simulink model "Modelo_Red_Mitigación_final"  (R2019b)
settings: Solver=VariableStepAuto  StartTime=0.0  StopTime=2.5  RelTol=1e-3
InitFcn:
  | Ts=20e-6;
undefined symbols (not defined in the file): D1, Delta, Ion, Lithium
libraries: powerlib x371, powerlib_meascontrol x286, simulink x50, simulink_extras x20, electricdrivelib x16
(part 1 of 11)
settings Model: Creator=ASUS  LastModifiedBy=mance
settings SolverCC: AlgebraicLoopSolver=LineSearch

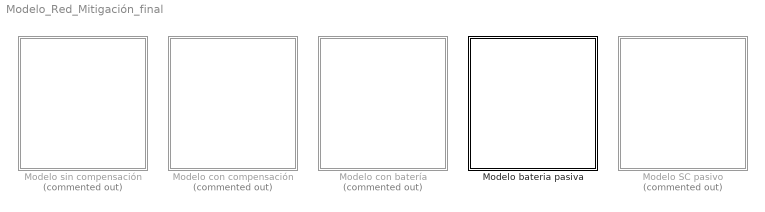
== system Modelo_Red_Mitigación_final ==
  Modelo SC pasivo : Subsystem  Commented=on
  Modelo bateria pasiva : Subsystem
  "Modelo con batería " : Subsystem  Commented=on
  Modelo con compensación : Subsystem  Commented=on
  Modelo sin compensación : Subsystem  Commented=on

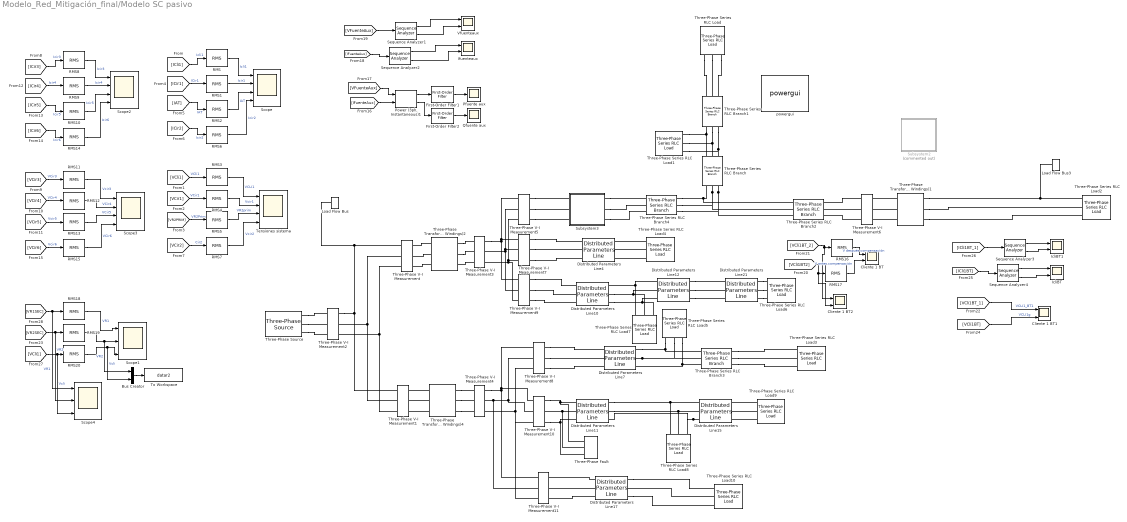
== system Modelo_Red_Mitigación_final/Modelo SC pasivo ==
  Bus Creator : BusCreator  Inputs=2
  Cliente 1 BT : Scope  NumInputPorts=2
  Cliente 1 BT1 : Scope  NumInputPorts=3
  Cliente 1 BT2 : Scope  NumInputPorts=2
  Distributed Parameters Line10 : powerlib/Elements/Distributed Parameters Line  Phases=3  Frequency=60  Resistance=[0.213 0.639]  Inductance=[0.78e-3 2.35e-3]  Capacitance=[15e-9 15e-9]  Length=3  x1=[-2e-05 2.82954479507891e-09 32197.4628123599 -19329.1003175042;-1e-05 2.80813823558566e-09 32270.1028326165 -19207.5816752081]  x2=[-2e-05 2.77830767246127e-09 31710.0647284196 -19350.9504482248;-1e-05 2.75705345961333e-09 31782.7905850361 -19231.2690937948]  x3=[-2e-05 -1.24111133051853e-11 -137.606557855475 265.255923665155;-1e-05 -1.24858274424735e-11 -138.605568913231 264.73527545555]  x4=[-2e-05 2.72589848097641e-11 416.943661034301 -435.06441838885;-1e-05 2.72249332713776e-11 418.580848519875 -433.489489926912]  x5=1.78115131305569e-05  V1=ones(3,3)  V2=ones(3,3)  I1=ones(3,3)  I2=ones(3,3)  nHarmo=1  Measurements=None
      settings: SourceProductName=Simscape Electrical
  Distributed Parameters Line11 : powerlib/Elements/Distributed Parameters Line  Phases=3  Frequency=60  Resistance=[0.269 0.807]  Inductance=[0.85e-3 2.56e-3]  Capacitance=[15e-9 15e-9]  Length=18  x1=[-0.00012 9.28558517205125e-09 31499.5304856781 -20459.5850295864;-0.00011 9.33622831118938e-09 31576.4372823811 -20340.6894905972;-0.0001 9.38673876185742e-09 31652.8953080157 -20221.5048653861;-9e-05 9.43711580619005e-09 31728.9034759441 -20102.0328478305;-8e-05 9.48735872821797e-09 31804.460705922 -19982.2751358921;-7e-05 9.53746681387805e-09 31879.565924114 -19862.2334315932;-6e-05 9.58743935102346e-09 31954.2180631086 -19741.9094409921;-5e-05 9.63727562943386e-09 32028.4160619336 -19621.304874159;-4e-05 9.68697494082539e-09 32102.1588660714 -19500.4214451518;-3e-05 9.73653657886085e-09 32175.4454274734 -19379.2608719915;-2e-05 9.78595983915965e-09 32248.2747045753 -19257.8248766382;-1e-05 9.83524401930785e-09 32320.645662312 -19136.1151849661]  x2=[-0.00012 7.5254042731239e-09 29691.2836160491 -20133.8764409861;-0.00011 7.57085579555663e-09 29766.9753728049 -20021.8001304674;-0.0001 7.61619971937037e-09 29842.2440749513 -19909.4392658505;-9e-05 7.6614354001276e-09 29917.0886527534 -19796.795444032;-8e-05 7.70656219492916e-09 29991.5080425041 -19683.87026593;-7e-05 7.75157946242343e-09 30065.5011865392 -19570.6653364611;-6e-05 7.79648656281536e-09 30139.0670332523 -19457.182264518;-5e-05 7.84128285787568e-09 30212.2045371099 -19343.4226629463;-4e-05 7.88596771094986e-09 30284.9126586661 -19229.3881485218;-3e-05 7.93054048696724e-09 30357.1903645776 -19115.0803419274;-2e-05 7.97500055245001e-09 30429.0366276182 -19000.50086773;-1e-05 8.01934727552222e-09 30500.4504266936 -18885.6513543576]  x3=[-0.00012 1.82517240735292e-11 9.27297529817065 123.366608204449;-0.00011 1.80056496454053e-11 8.80782934901758 123.400689758644;-0.0001 1.77593193171444e-11 8.34255822111328 123.43301751589;-9e-05 1.75127365896455e-11 7.87716852699037 123.463591016737;-8e-05 1.72659049673952e-11 7.41166688086653 123.492409826668;-7e-05 1.70188279584172e-11 6.94605989855056 123.519473536105;-6e-05 1.67715090742226e-11 6.48035419734828 123.544781760411;-5e-05 1.65239518297602e-11 6.01455639596856 123.568334139902;-4e-05 1.62761597433665e-11 5.5486731144292 123.590130339845;-3e-05 1.60281363367154e-11 5.08271097396287 123.610170050469;-2e-05 1.57798851347687e-11 4.616676596923 123.628452986965;-1e-05 1.55314096657253e-11 4.15057660668964 123.644978889491]  x4=[-0.00012 1.97670884628206e-11 241.846087556996 -294.396448705046;-0.00011 2.02416146680514e-11 242.954214808572 -293.482620581729;-0.0001 2.07158531951328e-11 244.058889142975 -292.564621420748;-9e-05 2.11897973040857e-11 245.160094860337 -291.642464268904;-8e-05 2.16634402591152e-11 246.257816310088 -290.71616223209;-7e-05 2.21367753287064e-11 247.352037891177 -289.78572847511;-6e-05 2.26097957857204e-11 248.442744052292 -288.851176221485;-5e-05 2.30824949074893e-11 249.529919292085 -287.912518753273;-4e-05 2.35548659759124e-11 250.613548159388 -286.969769410873;-3e-05 2.40269022775511e-11 251.693615253439 -286.022941592841;-2e-05 2.44985971037248e-11 252.770105224091 -285.072048755695;-1e-05 2.49699437506059e-11 253.84300277204 -284.117104413728]  x5=0.000111541920370774  V1=ones(3,3)  V2=ones(3,3)  I1=ones(3,3)  I2=ones(3,3)  nHarmo=1  Measurements=None
      settings: SourceProductName=Simscape Electrical
  Distributed Parameters Line12 : powerlib/Elements/Distributed Parameters Line  Phases=3  Frequency=60  Resistance=[0.269 0.807]  Inductance=[0.85e-3 2.56e-3]  Capacitance=[15e-9 15e-9]  Length=6  x1=[-4e-05 2.82073076764042e-09 0 0;-3e-05 2.79954747134583e-09 31636.8882015929 -19470.3567828154;-2e-05 2.77832438728486e-09 31710.0647284196 -19350.9504482248;-1e-05 2.75706181708451e-09 31782.7905850361 -19231.2690937948]  x2=[-4e-05 2.78987730105737e-09 0 0;-3e-05 2.76958553508523e-09 30859.2103716023 -19384.6974111384;-2e-05 2.74925440717215e-09 30932.0694972323 -19268.2234546569;-1e-05 2.72888420626845e-09 31004.4890096864 -19151.4756540699]  x3=[-4e-05 -1.98992952470769e-11 0 0;-3e-05 -1.98837592301982e-11 -40.5630647731358 176.429249490701;-2e-05 -1.98679406210881e-11 -41.2278975530833 176.275076976282;-1e-05 -1.9851839644564e-11 -41.8921443933484 176.118399202833]  x4=[-4e-05 3.43143588294857e-11 0 0;-3e-05 3.42061237078561e-11 301.110986467072 -339.88208633785;-2e-05 3.40974024414932e-11 302.390168983809 -338.744512112722;-1e-05 3.39881965755668e-11 303.665053866903 -337.602123578264]  x5=3.71806401235912e-05  V1=ones(3,3)  V2=ones(3,3)  I1=ones(3,3)  I2=ones(3,3)  nHarmo=1  Measurements=None
      settings: SourceProductName=Simscape Electrical
  Distributed Parameters Line15 : powerlib/Elements/Distributed Parameters Line  Phases=3  Frequency=60  Resistance=[0.269 0.807]  Inductance=[0.85e-3 2.56e-3]  Capacitance=[15e-9 15e-9]  Length=12  x1=[-8e-05 7.70836321616229e-09 0 0;-7e-05 7.75338281960844e-09 0 0;-6e-05 7.79829223032257e-09 0 0;-5e-05 7.84309081004255e-09 30212.2045371099 -19343.4226629463;-4e-05 7.8877779220814e-09 30284.9126586661 -19229.3881485218;-3e-05 7.93235293133633e-09 30357.1903645776 -19115.0803419274;-2e-05 7.97681520429781e-09 30429.0366276182 -19000.50086773;-1e-05 8.02116410905851e-09 30500.4504266936 -18885.6513543576]  x2=[-8e-05 7.36763865817834e-09 0 0;-7e-05 7.41180338430477e-09 0 0;-6e-05 7.45586277229905e-09 0 0;-5e-05 7.49981619597974e-09 29831.7562384286 -19278.8102742345;-4e-05 7.5436630306714e-09 29904.2234811012 -19166.2104718515;-3e-05 7.58740265321346e-09 29976.2657185649 -19053.3382751932;-2e-05 7.63103444196906e-09 30047.8819269402 -18940.1952884233;-1e-05 7.67455777683391e-09 30119.0710884021 -18826.7831195541]  x3=[-8e-05 1.51035721072039e-11 0 0;-7e-05 1.51133669251181e-11 0 0;-6e-05 1.51229469486348e-11 0 0;-5e-05 1.51323120416007e-11 86.3804979587916 -15.5854425693932;-4e-05 1.51414620709169e-11 86.4386397248316 -15.2596857835742;-3e-05 1.51503969065415e-11 86.4955530064687 -14.9337121238428;-2e-05 1.51591164214905e-11 86.5512369948392 -14.6075262230064;-1e-05 1.51676204918403e-11 86.6056908985504 -14.2811327168884]  x4=[-8e-05 2.09154201224528e-11 0 0;-7e-05 2.11216506844416e-11 0 0;-6e-05 2.13275810610214e-11 0 0;-5e-05 2.15332083254655e-11 162.002074810409 -147.043074965172;-4e-05 2.17385295553554e-11 162.555261626192 -146.431298074321;-3e-05 2.1943541832622e-11 163.10613817189 -145.817440070599;-2e-05 2.2148242243587e-11 163.654696618329 -145.201509678285;-1e-05 2.23526278790045e-11 164.200929169278 -144.583515651115]  x5=7.43612802471824e-05  V1=ones(3,3)  V2=ones(3,3)  I1=ones(3,3)  I2=ones(3,3)  nHarmo=1  Measurements=None
      settings: SourceProductName=Simscape Electrical
  Distributed Parameters Line17 : powerlib/Elements/Distributed Parameters Line  Phases=3  Frequency=60  Resistance=[0.213 0.639]  Inductance=[0.78e-3 2.35e-3]  Capacitance=[15e-9 15e-9]  Length=18  x1=[-0.00011 9.33622831118938e-09 31576.4372823811 -20340.6894905972;-0.0001 9.38673876185742e-09 31652.8953080157 -20221.5048653861;-9e-05 9.43711580619005e-09 31728.9034759441 -20102.0328478305;-8e-05 9.48735872821797e-09 31804.460705922 -19982.2751358921;-7e-05 9.53746681387805e-09 31879.565924114 -19862.2334315932;-6e-05 9.58743935102346e-09 31954.2180631086 -19741.9094409921;-5e-05 9.63727562943386e-09 32028.4160619336 -19621.304874159;-4e-05 9.68697494082539e-09 32102.1588660714 -19500.4214451518;-3e-05 9.73653657886085e-09 32175.4454274734 -19379.2608719915;-2e-05 9.78595983915965e-09 32248.2747045753 -19257.8248766382;-1e-05 9.83524401930785e-09 32320.645662312 -19136.1151849661]  x2=[-0.00011 8.47298600701393e-09 30855.9731260701 -20386.4569187283;-0.0001 8.52187570130671e-09 30932.6088101304 -20269.9880477362;-9e-05 8.57064428088256e-09 31008.80487335 -20153.2310953462;-8e-05 8.619291052632e-09 31084.5602328142 -20036.187720933;-7e-05 8.66781532517675e-09 31159.8738118716 -19918.8595879421;-6e-05 8.71621640887946e-09 31234.7445401497 -19801.2483638659;-5e-05 8.76449361585362e-09 31309.1713535696 -19683.3557202204;-4e-05 8.81264625997324e-09 31383.1531943615 -19565.1833325208;-3e-05 8.86067365688267e-09 31456.6890110797 -19446.7328802585;-2e-05 8.90857512400629e-09 31529.7777586176 -19328.0060468765;-1e-05 8.95634998055821e-09 31602.4183982221 -19209.0045197459]  x3=[-0.00011 1.41778636431536e-11 65.9616338670945 -5.20882786217487;-0.0001 1.4124703549912e-11 65.9808019085836 -4.96012193546151;-9e-05 1.40713427133679e-11 65.9990322168288 -4.71134551443619;-8e-05 1.40177818918968e-11 66.0163245327368 -4.46250213476252;-7e-05 1.39640218467166e-11 66.0326786105459 -4.21359533305574;-6e-05 1.39100633418766e-11 66.0480942178282 -3.96462864683246;-5e-05 1.38559071442464e-11 66.0625711354938 -3.71560561446039;-4e-05 1.38015540235056e-11 66.0761091577937 -3.46652977510802;-3e-05 1.37470047521323e-11 66.0887080923227 -3.21740466869437;-2e-05 1.36922601053925e-11 66.100367760022 -2.96823383583863;-1e-05 1.36373208613286e-11 66.1110879951819 -2.71902081780988]  x4=[-0.00011 2.75162896081253e-11 202.338595789073 -174.305940383283;-0.0001 2.78192962474476e-11 202.994274307036 -173.541905018224;-9e-05 2.81219075129921e-11 203.647067827032 -172.775403238559;-8e-05 2.84241191039828e-11 204.29696707142 -172.006445937975;-7e-05 2.87259267253241e-11 204.943962803694 -171.235044045056;-6e-05 2.90273260876617e-11 205.588045828612 -170.461208523132;-5e-05 2.93283129074434e-11 206.229206992328 -169.684950370118;-4e-05 2.96288829069803e-11 206.867437182524 -168.906280618361;-3e-05 2.99290318145074e-11 207.502727328535 -168.125210334482;-2e-05 3.02287553642444e-11 208.135068401482 -167.341750619217;-1e-05 3.05280492964561e-11 208.764451414399 -166.555912607264]  x5=0.000106869078783341  V1=ones(3,3)  V2=ones(3,3)  I1=ones(3,3)  I2=ones(3,3)  nHarmo=1  Measurements=None
      settings: SourceProductName=Simscape Electrical
  Distributed Parameters Line21 : powerlib/Elements/Distributed Parameters Line  Phases=3  Frequency=60  Resistance=[0.269 0.807]  Inductance=[0.85e-3 2.56e-3]  Capacitance=[15e-9 15e-9]  Length=3  x1=[-2e-05 2.75107077336082e-09 30932.0694972323 -19268.2234546569;-1e-05 2.73070189698126e-09 31004.4890096864 -19151.4756540699]  x2=[-2e-05 2.75481069609383e-09 30542.7078876513 -19225.7498451882;-1e-05 2.73620987629515e-09 30614.9700455945 -19110.470201633]  x3=[-2e-05 -9.10606690504655e-11 -43.7912955115461 177.913060929838;-1e-05 -9.08089001289591e-11 -44.4616991754304 177.746707756957]  x4=[-2e-05 1.0010549597789e-10 301.055370570621 -339.730088442752;-1e-05 9.97734452086656e-11 302.333980465362 -338.59272496423]  x5=1.85903200617956e-05  V1=ones(3,3)  V2=ones(3,3)  I1=ones(3,3)  I2=ones(3,3)  nHarmo=1  Measurements=None
      settings: SourceProductName=Simscape Electrical
  Distributed Parameters Line4 : powerlib/Elements/Distributed Parameters Line  Phases=3  Frequency=60  Resistance=[0.213 0.639]  Inductance=[0.78e-3 2.35e-3]  Capacitance=[15e-9 15e-9]  Length=9  x1=[-6e-05 2.91476585835731e-09 31902.3371803933 -19812.410581904;-5e-05 2.89352197491375e-09 31976.8013302996 -19692.0010999389;-4e-05 2.87223696811809e-09 32050.8110190781 -19571.3117510499;-3e-05 2.8509111404774e-09 32124.3651948874 -19450.3442504996;-2e-05 2.82954479507891e-09 32197.4628123599 -19329.1003175042;-1e-05 2.80813823558566e-09 32270.1028326165 -19207.5816752081]  x2=[-6e-05 2.8671151692512e-09 31242.7818227804 -19858.7298296781;-5e-05 2.84653547177567e-09 31317.4252785941 -19740.8064777932;-4e-05 2.82591531873026e-09 31391.6236444732 -19622.6025653518;-3e-05 2.80525500317299e-09 31465.3758658949 -19504.1197722932;-2e-05 2.78455481873268e-09 31538.6808946767 -19385.3597825202;-1e-05 2.76381505960478e-09 31611.537688992 -19266.3242838751]  x3=[-6e-05 -8.71600142727094e-12 9.18504689485535 67.3502715851573;-5e-05 -8.7408702746565e-12 8.93107768424118 67.3844197159342;-4e-05 -8.7656148949275e-12 8.67698154324412 67.4176101649512;-3e-05 -8.7902349364081e-12 8.42276208313279 67.4498424604985;-2e-05 -8.81473004919303e-12 8.16842291692843 67.4811161444838;-1e-05 -8.8390998851525e-12 7.91396765935357 67.5114307724389]  x4=[-6e-05 2.55850021468679e-11 264.979509807935 -241.826806008615;-5e-05 2.55047562310245e-11 265.889290256423 -240.826140710092;-4e-05 2.54241478361401e-11 266.795291829549 -239.82205273904;-3e-05 2.53431781078385e-11 267.697501651025 -238.814556365771;-2e-05 2.52618481968787e-11 268.595906898453 -237.803665909039;-1e-05 2.51801592591388e-11 269.490494803506 -236.789395735835]  x5=5.34345393916706e-05  V1=ones(3,3)  V2=ones(3,3)  I1=ones(3,3)  I2=ones(3,3)  nHarmo=1  Measurements=None
      settings: SourceProductName=Simscape Electrical
  Distributed Parameters Line7 : powerlib/Elements/Distributed Parameters Line  Phases=3  Frequency=60  Resistance=[0.213 0.639]  Inductance=[0.78e-3 2.35e-3]  Capacitance=[15e-9 15e-9]  Length=4.4  x1=[-3e-05 9.73653657886085e-09 0 0;-2e-05 9.78595983915965e-09 32248.2747045753 -19257.8248766382;-1e-05 9.83524401930785e-09 32320.645662312 -19136.1151849661]  x2=[-3e-05 9.36426318599823e-09 0 0;-2e-05 9.41286833190097e-09 31944.5740855089 -19310.7767627906;-1e-05 9.46133970010929e-09 32017.1468248096 -19190.2116164852]  x3=[-3e-05 1.42465334878302e-11 0 0;-2e-05 1.40327784500841e-11 2.66918275739884 49.6416949019883;-1e-05 1.38188239754946e-11 2.48201945237274 49.6514047008997]  x4=[-3e-05 3.31318337680973e-11 0 0;-2e-05 3.35913918708071e-11 277.490011326945 -219.052715302811;-1e-05 3.40504725654836e-11 278.313846778578 -218.005048471527]  x5=2.61235525914834e-05  V1=ones(3,3)  V2=ones(3,3)  I1=ones(3,3)  I2=ones(3,3)  nHarmo=1  Measurements=None
      settings: SourceProductName=Simscape Electrical
  First-Order Filter1 : powerlib_meascontrol/Filters/First-Order Filter  FilterType=Lowpass  Tc=10e-3  Ts=0  Initialize=on  Vac_Init=[0, 0, 60]  Vdc_Init=0  PlotResponse=off  FreqRange="[0,  200,  1]"
      settings: SourceProductName=Simscape Electrical
  First-Order Filter2 : powerlib_meascontrol/Filters/First-Order Filter  FilterType=Lowpass  Tc=10e-3  Ts=0  Initialize=on  Vac_Init=[0, 0, 60]  Vdc_Init=0  PlotResponse=off  FreqRange="[0,  200,  1]"
      settings: SourceProductName=Simscape Electrical
  IcliBT : Scope  NumInputPorts=2
  IcliBT1 : Scope  NumInputPorts=2
  Ifuenteaux : Scope  NumInputPorts=2
  Load Flow Bus : powerlib/Measurements/Load Flow Bus  LConnTagsString=a  Phases=single  Connectors=on one side  ID=BUS_1  Vbase=115e3  Vref=1.05  Vangle=0  VLF=1  VLFb=1  VLFc=1  angleLF=0  angleLFb=0  angleLFc=0
      settings: SourceProductName=Simscape Electrical
  Load Flow Bus3 : powerlib/Measurements/Load Flow Bus  LConnTagsString=a  Phases=single  Connectors=on one side  ID=BUS_4  Vbase=440  Vref=1  Vangle=0  VLF=0.9785  VLFb=1  VLFc=1  angleLF=28.33  angleLFb=0  angleLFc=0
      settings: SourceProductName=Simscape Electrical
  "Pfuente aux " : Scope
  "Power (3ph, Instantaneous)1" : powerlib_meascontrol/Measurements/Power (3ph, Instantaneous)
      settings: SourceProductName=Simscape Electrical
  Qfuente aux : Scope
  RMS{,1..20} (21 alike) : powerlib_meascontrol/Measurements/RMS  TrueRMS=on  Freq=60  RMSInit=120  Ts=0
      settings: SourceProductName=Simscape Electrical
  Scope : Scope  NumInputPorts=4
  Scope1 : Scope  NumInputPorts=3
  Scope2 : Scope  NumInputPorts=4
  Scope3 : Scope  NumInputPorts=4
  Scope4 : Scope  NumInputPorts=3
  Sequence Analyzer{1..4} (4 alike) : powerlib_meascontrol/Measurements/Sequence Analyzer  Freq=60  n=1  seq=Positive Negative Zero  InInit=[1, 0]  Ts=0
      settings: SourceProductName=Simscape Electrical  SourceProductBaseCode=PS
  Subsystem2 : Subsystem  Commented=on
  Subsystem3 : Subsystem
  Tensiones sistema : Scope  NumInputPorts=4
  Three-Phase Series RLC Branch : powerlib/Elements/Three-Phase Series RLC Branch  LConnTagsString=A|B|C  RConnTagsString=A|B|C  BranchType=RL  Resistance=0.213  Inductance=0.78e-3  Capacitance=1e-6  Measurements=None
      settings: SourceProductName=Simscape Electrical
  Three-Phase Series RLC Branch1 : powerlib/Elements/Three-Phase Series RLC Branch  LConnTagsString=A|B|C  RConnTagsString=A|B|C  BranchType=RL  Resistance=0.213  Inductance=0.78e-3  Capacitance=1e-6  Measurements=None
      settings: SourceProductName=Simscape Electrical
  Three-Phase Series RLC Branch2 : powerlib/Elements/Three-Phase Series RLC Branch  LConnTagsString=A|B|C  RConnTagsString=A|B|C  BranchType=RL  Resistance=0.213*1.7  Inductance=0.78e-3*1.7  Capacitance=1e-6  Measurements=None
      settings: SourceProductName=Simscape Electrical
  Three-Phase Series RLC Branch3 : powerlib/Elements/Three-Phase Series RLC Branch  LConnTagsString=A|B|C  RConnTagsString=A|B|C  BranchType=RL  Resistance=0.213*2.2  Inductance=0.78e-3*2.2  Capacitance=1e-6  Measurements=None
      settings: SourceProductName=Simscape Electrical
  Three-Phase Series RLC Branch4 : powerlib/Elements/Three-Phase Series RLC Branch  LConnTagsString=A|B|C  RConnTagsString=A|B|C  BranchType=RL  Resistance=0.213*7  Inductance=0.78e-3*7  Capacitance=1e-6  Measurements=None
      settings: SourceProductName=Simscape Electrical
  Three-Phase Series RLC Load : powerlib/Elements/Three-Phase Series RLC Load  LConnTagsString=A|B|C  Configuration=Y (grounded)  NominalVoltage=34.5e3  Vabc=[1e3 1e3 1e3]  Vabcp=[1e3 1e3 1e3]  NominalFrequency=60  UnbalancedPower=off  ActivePower=0.5e6  InductivePower=0.1e6  CapacitivePower=0  Pabc=[10e3 9e3 11e3]  QLabc=[100 90 110]  QCabc=[100 90 110]  Pabcp=[10e3 9e3 11e3]  QLabcp=[100 90 110]  QCabcp=[100 90 110]  Measurements=None  LoadType=constant Z
      settings: SourceProductName=Simscape Electrical
  Three-Phase Series RLC Load1 : powerlib/Elements/Three-Phase Series RLC Load  LConnTagsString=A|B|C  Configuration=Y (grounded)  NominalVoltage=34.5e3  Vabc=[1e3 1e3 1e3]  Vabcp=[1e3 1e3 1e3]  NominalFrequency=60  UnbalancedPower=off  ActivePower=2.5e6  InductivePower=1e6  CapacitivePower=0  Pabc=[10e3 9e3 11e3]  QLabc=[100 90 110]  QCabc=[100 90 110]  Pabcp=[10e3 9e3 11e3]  QLabcp=[100 90 110]  QCabcp=[100 90 110]  Measurements=None  LoadType=constant Z
      settings: SourceProductName=Simscape Electrical
  Three-Phase Series RLC Load10 : powerlib/Elements/Three-Phase Series RLC Load  LConnTagsString=A|B|C  Configuration=Y (grounded)  NominalVoltage=34.5e3  Vabc=[1e3 1e3 1e3]  Vabcp=[1e3 1e3 1e3]  NominalFrequency=60  UnbalancedPower=off  ActivePower=3.4e6  InductivePower=1.1e6  CapacitivePower=0  Pabc=[10e3 9e3 11e3]  QLabc=[100 90 110]  QCabc=[100 90 110]  Pabcp=[10e3 9e3 11e3]  QLabcp=[100 90 110]  QCabcp=[100 90 110]  Measurements=None  LoadType=constant Z
      settings: SourceProductName=Simscape Electrical
  Three-Phase Series RLC Load2 : powerlib/Elements/Three-Phase Series RLC Load  LConnTagsString=A|B|C  Configuration=Y (grounded)  NominalVoltage=440  Vabc=[1e3 1e3 1e3]  Vabcp=[1e3 1e3 1e3]  NominalFrequency=60  UnbalancedPower=off  ActivePower=6.5e6  InductivePower=3e6  CapacitivePower=0  Pabc=[10e3 9e3 11e3]  QLabc=[100 90 110]  QCabc=[100 90 110]  Pabcp=[10e3 9e3 11e3]  QLabcp=[100 90 110]  QCabcp=[100 90 110]  Measurements=None  LoadType=constant Z
      settings: SourceProductName=Simscape Electrical
  Three-Phase Series RLC Load3 : powerlib/Elements/Three-Phase Series RLC Load  LConnTagsString=A|B|C  Configuration=Y (grounded)  NominalVoltage=34.5e3  Vabc=[1e3 1e3 1e3]  Vabcp=[1e3 1e3 1e3]  NominalFrequency=60  UnbalancedPower=off  ActivePower=3e6  InductivePower=0.7e6  CapacitivePower=0  Pabc=[10e3 9e3 11e3]  QLabc=[100 90 110]  QCabc=[100 90 110]  Pabcp=[10e3 9e3 11e3]  QLabcp=[100 90 110]  QCabcp=[100 90 110]  Measurements=None  LoadType=constant Z
      settings: SourceProductName=Simscape Electrical
  Three-Phase Series RLC Load4 : powerlib/Elements/Three-Phase Series RLC Load  LConnTagsString=A|B|C  Configuration=Y (grounded)  NominalVoltage=34.5e3  Vabc=[1e3 1e3 1e3]  Vabcp=[1e3 1e3 1e3]  NominalFrequency=60  UnbalancedPower=off  ActivePower=6.2e6  InductivePower=2e6  CapacitivePower=0  Pabc=[10e3 9e3 11e3]  QLabc=[100 90 110]  QCabc=[100 90 110]  Pabcp=[10e3 9e3 11e3]  QLabcp=[100 90 110]  QCabcp=[100 90 110]  Measurements=None  LoadType=constant Z
      settings: SourceProductName=Simscape Electrical
  Three-Phase Series RLC Load5 : powerlib/Elements/Three-Phase Series RLC Load  LConnTagsString=A|B|C  Configuration=Y (grounded)  NominalVoltage=34.5e3  Vabc=[1e3 1e3 1e3]  Vabcp=[1e3 1e3 1e3]  NominalFrequency=60  UnbalancedPower=off  ActivePower=3e6  InductivePower=0.7e6  CapacitivePower=0  Pabc=[10e3 9e3 11e3]  QLabc=[100 90 110]  QCabc=[100 90 110]  Pabcp=[10e3 9e3 11e3]  QLabcp=[100 90 110]  QCabcp=[100 90 110]  Measurements=None  LoadType=constant Z
      settings: SourceProductName=Simscape Electrical
  Three-Phase Series RLC Load6 : powerlib/Elements/Three-Phase Series RLC Load  LConnTagsString=A|B|C  Configuration=Y (grounded)  NominalVoltage=34.5e3  Vabc=[1e3 1e3 1e3]  Vabcp=[1e3 1e3 1e3]  NominalFrequency=60  UnbalancedPower=off  ActivePower=9.4e6  InductivePower=4.2e6  CapacitivePower=0  Pabc=[10e3 9e3 11e3]  QLabc=[100 90 110]  QCabc=[100 90 110]  Pabcp=[10e3 9e3 11e3]  QLabcp=[100 90 110]  QCabcp=[100 90 110]  Measurements=None  LoadType=constant Z
      settings: SourceProductName=Simscape Electrical
  Three-Phase Series RLC Load7 : powerlib/Elements/Three-Phase Series RLC Load  LConnTagsString=A|B|C  Configuration=Y (grounded)  NominalVoltage=34.5e3  Vabc=[1e3 1e3 1e3]  Vabcp=[1e3 1e3 1e3]  NominalFrequency=60  UnbalancedPower=off  ActivePower=4.4e6  InductivePower=0.8e6  CapacitivePower=0  Pabc=[10e3 9e3 11e3]  QLabc=[100 90 110]  QCabc=[100 90 110]  Pabcp=[10e3 9e3 11e3]  QLabcp=[100 90 110]  QCabcp=[100 90 110]  Measurements=None  LoadType=constant Z
      settings: SourceProductName=Simscape Electrical
  Three-Phase Series RLC Load8 : powerlib/Elements/Three-Phase Series RLC Load  LConnTagsString=A|B|C  Configuration=Y (grounded)  NominalVoltage=34.5e3  Vabc=[1e3 1e3 1e3]  Vabcp=[1e3 1e3 1e3]  NominalFrequency=60  UnbalancedPower=off  ActivePower=5e6  InductivePower=2.5e6  CapacitivePower=0  Pabc=[10e3 9e3 11e3]  QLabc=[100 90 110]  QCabc=[100 90 110]  Pabcp=[10e3 9e3 11e3]  QLabcp=[100 90 110]  QCabcp=[100 90 110]  Measurements=None  LoadType=constant Z
      settings: SourceProductName=Simscape Electrical
  Three-Phase Series RLC Load9 : powerlib/Elements/Three-Phase Series RLC Load  LConnTagsString=A|B|C  Configuration=Y (grounded)  NominalVoltage=34.5e3  Vabc=[1e3 1e3 1e3]  Vabcp=[1e3 1e3 1e3]  NominalFrequency=60  UnbalancedPower=off  ActivePower=2.3e6  InductivePower=1.2e6  CapacitivePower=0  Pabc=[10e3 9e3 11e3]  QLabc=[100 90 110]  QCabc=[100 90 110]  Pabcp=[10e3 9e3 11e3]  QLabcp=[100 90 110]  QCabcp=[100 90 110]  Measurements=None  LoadType=constant Z
      settings: SourceProductName=Simscape Electrical
  Three-Phase V-I Measurement : powerlib/Measurements/Three-Phase V-I Measurement  VoltageMeasurement=phase-to-ground  SetLabelV=on  LabelV=VR2PRIM  Vpu=off  VpuLL=off  CurrentMeasurement=yes  SetLabelI=on  LabelI=IR2PRIM  Ipu=off  Pbase=100e6  Vbase=500e3  OutputType=Complex  PhasorSimulation=off  PSBequivalent=0
      settings: SourceProductName=Simscape Electrical
  Three-Phase V-I Measurement1 : powerlib/Measurements/Three-Phase V-I Measurement  VoltageMeasurement=phase-to-ground  SetLabelV=on  LabelV=VR1PRIM  Vpu=off  VpuLL=off  CurrentMeasurement=yes  SetLabelI=on  LabelI=IR1PRIM  Ipu=off  Pbase=100e6  Vbase=500e3  OutputType=Complex  PhasorSimulation=off  PSBequivalent=0
      settings: SourceProductName=Simscape Electrical
  Three-Phase V-I Measurement10 : powerlib/Measurements/Three-Phase V-I Measurement  VoltageMeasurement=phase-to-ground  SetLabelV=on  LabelV=VCir5  Vpu=off  VpuLL=off  CurrentMeasurement=yes  SetLabelI=on  LabelI=ICir5  Ipu=off  Pbase=100e6  Vbase=500e3  OutputType=Complex  PhasorSimulation=off  PSBequivalent=0
      settings: SourceProductName=Simscape Electrical
  Three-Phase V-I Measurement11 : powerlib/Measurements/Three-Phase V-I Measurement  VoltageMeasurement=phase-to-ground  SetLabelV=on  LabelV=VCir6  Vpu=off  VpuLL=off  CurrentMeasurement=yes  SetLabelI=on  LabelI=ICir6  Ipu=off  Pbase=100e6  Vbase=500e3  OutputType=Complex  PhasorSimulation=off  PSBequivalent=0
      settings: SourceProductName=Simscape Electrical
  Three-Phase V-I Measurement2 : powerlib/Measurements/Three-Phase V-I Measurement  VoltageMeasurement=phase-to-ground  SetLabelV=on  LabelV=VAT  Vpu=off  VpuLL=off  CurrentMeasurement=yes  SetLabelI=on  LabelI=IAT  Ipu=off  Pbase=100e6  Vbase=500e3  OutputType=Complex  PhasorSimulation=off  PSBequivalent=0
      settings: SourceProductName=Simscape Electrical
  Three-Phase V-I Measurement3 : powerlib/Measurements/Three-Phase V-I Measurement  VoltageMeasurement=phase-to-ground  SetLabelV=on  LabelV=VR2SEC  Vpu=off  VpuLL=off  CurrentMeasurement=yes  SetLabelI=on  LabelI=IR2SEC  Ipu=off  Pbase=100e6  Vbase=500e3  OutputType=Complex  PhasorSimulation=off  PSBequivalent=0
      settings: SourceProductName=Simscape Electrical
  Three-Phase V-I Measurement4 : powerlib/Measurements/Three-Phase V-I Measurement  VoltageMeasurement=phase-to-ground  SetLabelV=on  LabelV=VR1SEC  Vpu=off  VpuLL=off  CurrentMeasurement=yes  SetLabelI=on  LabelI=IR1SEC  Ipu=off  Pbase=100e6  Vbase=500e3  OutputType=Complex  PhasorSimulation=off  PSBequivalent=0
      settings: SourceProductName=Simscape Electrical
  Three-Phase V-I Measurement5 : powerlib/Measurements/Three-Phase V-I Measurement  VoltageMeasurement=phase-to-ground  SetLabelV=on  LabelV=VCir1  Vpu=off  VpuLL=off  CurrentMeasurement=yes  SetLabelI=on  LabelI=ICir1  Ipu=off  Pbase=100e6  Vbase=500e3  OutputType=Complex  PhasorSimulation=off  PSBequivalent=0
      settings: SourceProductName=Simscape Electrical
  Three-Phase V-I Measurement6 : powerlib/Measurements/Three-Phase V-I Measurement  VoltageMeasurement=phase-to-ground  SetLabelV=on  LabelV=VCli1  Vpu=off  VpuLL=off  CurrentMeasurement=yes  SetLabelI=on  LabelI=ICli1  Ipu=off  Pbase=100e6  Vbase=500e3  OutputType=Complex  PhasorSimulation=off  PSBequivalent=0
      settings: SourceProductName=Simscape Electrical
  Three-Phase V-I Measurement7 : powerlib/Measurements/Three-Phase V-I Measurement  VoltageMeasurement=phase-to-ground  SetLabelV=on  LabelV=VCir2  Vpu=off  VpuLL=off  CurrentMeasurement=yes  SetLabelI=on  LabelI=ICir2  Ipu=off  Pbase=100e6  Vbase=500e3  OutputType=Complex  PhasorSimulation=off  PSBequivalent=0
      settings: SourceProductName=Simscape Electrical
  Three-Phase V-I Measurement8 : powerlib/Measurements/Three-Phase V-I Measurement  VoltageMeasurement=phase-to-ground  SetLabelV=on  LabelV=VCir4  Vpu=off  VpuLL=off  CurrentMeasurement=yes  SetLabelI=on  LabelI=ICir4  Ipu=off  Pbase=100e6  Vbase=500e3  OutputType=Complex  PhasorSimulation=off  PSBequivalent=0
      settings: SourceProductName=Simscape Electrical
  Three-Phase V-I Measurement9 : powerlib/Measurements/Three-Phase V-I Measurement  VoltageMeasurement=phase-to-ground  SetLabelV=on  LabelV=VCir3  Vpu=off  VpuLL=off  CurrentMeasurement=yes  SetLabelI=on  LabelI=ICir3  Ipu=off  Pbase=100e6  Vbase=500e3  OutputType=Complex  PhasorSimulation=off  PSBequivalent=0
      settings: SourceProductName=Simscape Electrical
  Three-Phase Fault : powerlib/Elements/Three-Phase Fault  InitialStates=0  FaultA=on  FaultB=on  FaultC=on  GroundFault=off  SwitchTimes=[0.1,0.8,0.9,1.6,1.7,2.4]  External=off  SwitchStatus=NaN  FaultResistance=0.3  GroundResistance=0.01  SnubberResistance=1e6  SnubberCapacitance=inf  Measurements=None
      settings: SourceProductName=Simscape Electrical
  Three-Phase Source : powerlib/Electrical Sources/Three-Phase Source  InternalConnection=Yg  VoltagePhases=off  Voltage=(115000)*1.39942  PhaseAngle=16.7311  Voltage_phases=[25e3 25e3 25e3]/sqrt(3)  PhaseAngles_phases=[0 -120 +120]  Frequency=60  NonIdealSource=on  SpecifyImpedance=on  Resistance=0.8929  Inductance=16.58e-3  ShortCircuitLevel=100e6  BaseVoltage=115e3  XRratio=5.946  BusType=swing  Pref=10e3  Qref=0  Prefabc=[10e3, 10e3, 10e3]  Qrefabc=[0, 0, 0]  Qmin=-inf  Qmax=inf
      settings: SourceProductName=Simscape Electrical
  Three-Phase Transformer Inductance Matrix Type (Two Windings)1 : powerlib/Elements/Three-Phase Transformer Inductance Matrix Type (Two Windings)  CoreType=Three-limb or five-limb core  Winding1Connection=Yg  Winding2Connection=Yg  AutoTransformer=off  Measurements=None  NominalPower=[10e6, 60]  VLLnom=[34.5e3, 440]  WindingResistances=[0.01, 0.01]  NoLoadIexcPos=2  NoLoadPlossPos=1000  ShortCircuitReactancePos=0.06  ShortCircuitReactancePosAuto=0.06  NoLoadIexcZero=100  NoLoadPlossZero=500000  ShortCircuitReactanceZero=0.03  ShortCircuitReactanceZeroAuto=0.03
      settings: SourceProductName=Simscape Electrical  SourceProductBaseCode=PS
  Three-Phase Transformer Inductance Matrix Type (Two Windings)2 : powerlib/Elements/Three-Phase Transformer Inductance Matrix Type (Two Windings)  CoreType=Three single-phase cores  Winding1Connection=Delta (D1)  Winding2Connection=Y  AutoTransformer=off  Measurements=None  NominalPower=[40e6, 60]  VLLnom=[115e3, 34.5e3]  WindingResistances=[0.006, 0.006]  NoLoadIexcPos=2  NoLoadPlossPos=16600  ShortCircuitReactancePos=0.1056  ShortCircuitReactancePosAuto=0.06  NoLoadIexcZero=100  NoLoadPlossZero=500000  ShortCircuitReactanceZero=0.1056  ShortCircuitReactanceZeroAuto=0.03
      settings: SourceProductName=Simscape Electrical  SourceProductBaseCode=PS
  Three-Phase Transformer Inductance Matrix Type (Two Windings)4 : powerlib/Elements/Three-Phase Transformer Inductance Matrix Type (Two Windings)  CoreType=Three single-phase cores  Winding1Connection=Delta (D1)  Winding2Connection=Y  AutoTransformer=off  Measurements=None  NominalPower=[30e6, 60]  VLLnom=[115e3, 34.5e3]  WindingResistances=[0.006, 0.006]  NoLoadIexcPos=2  NoLoadPlossPos=14300  ShortCircuitReactancePos=0.0912  ShortCircuitReactancePosAuto=0.06  NoLoadIexcZero=100  NoLoadPlossZero=500000  ShortCircuitReactanceZero=0.0912  ShortCircuitReactanceZeroAuto=0.03
      settings: SourceProductName=Simscape Electrical  SourceProductBaseCode=PS
  To Workspace : ToWorkspace  VariableName=datar2  SaveFormat=Timeseries  SampleTime=-1
  Vfuenteaux : Scope  NumInputPorts=2
  powergui : powerlib/powergui  Priority=1  SimulationMode=Discrete  SampleTime=10e-6  frequency=60  Iterations=50  frequencyindice=0  Pbase=100e6  ErrMax=0.0001  UnitsV=kV  UnitsW=MW  buscounter=0  FunctionMessages=off  echomessages=off  EnableUseOfTLC=off  CurrentSourceSwitches=off  DisableSnubberDevices=off  DisableRonSwitches=off  DisableVfSwitches=off  DisplayEquations=off  AutomaticDiscreteSolvers=off  SolverType=Tustin/Backward Euler (TBE)  Interpol=off  ExternalGateDelay=off  methode=off  Ts=100  x0status=blocks  SPID=on  SwTol=0  HookPort=off  NonlinearTolerance=1e-4  nMaxIteration=100  ContinueOnMaxIteration=off  RestoreLinks=warning  ResistiveCurrentMeasurement=off  Frange=[0:2:500]  Ylog=off  Xlog=on  ShowGrid=off  save=off  variable=ZData  structure=0  ZoomFFT=off  StartTime=0.0  cycles=1  DisplayStyle=1  fundamental=60  FreqAxis=off  MaxFrequency=1000  frequencyindicesteady=1  RmsSteady=1  display=off
      settings: SourceProductName=Simscape Electrical
  wires:
  RMS1/1 -> Scope/2  "Icir1"
  Sequence Analyzer4/2 -> IcliBT/2
  RMS5/1 -> Tensiones sistema/3  "VR2prim"
  [VCli1] -> RMS3/1  "VCli1"
  "Power (3ph, Instantaneous)1"/2 -> First-Order Filter2/1
  RMS13/1 -> Scope3/3  "VCir5"
  [ICir5] -> RMS10/1  "Icir5"
  Sequence Analyzer1/2 -> Vfuenteaux/2
  [ICir2] -> RMS6/1  "Icir2"
  RMS7/1 -> Tensiones sistema/4  "Vcir2"
  Sequence Analyzer3/1 -> IcliBT1/1
  Sequence Analyzer4/1 -> IcliBT/1
  RMS9/1 -> Scope2/2  "Icir4"
  [VCir3] -> RMS11/1  "VCir3"
  [VFuenteAux] -> Sequence Analyzer1/1
  [VCir5] -> RMS13/1  "Vcir5"
  [VCli1BT2] -> Cliente 1 BT2/2, RMS17/1
  [ICir1] -> RMS1/1  "ICir1"
  [VCir6] -> RMS15/1  "Vcir6"
  [ICli1BT] -> Sequence Analyzer4/1
  First-Order Filter1/1 -> "Pfuente aux "/1
  RMS3/1 -> Tensiones sistema/1  "VCLI1"
  [VCli1BT] -> Cliente 1 BT1/3  "VCLI1g"
  Sequence Analyzer3/2 -> IcliBT1/2
  Sequence Analyzer2/1 -> Ifuenteaux/1
  [VCli1BT_1] -> Cliente 1 BT1/1  "VCLI1_BT1"
  RMS17/1 -> Cliente 1 BT/2  "V antes compensación"
  RMS16/1 -> Cliente 1 BT/1  "V después compensación"
  [VCir2] -> RMS7/1  "Cir2"
  [ICli1BT_1] -> Sequence Analyzer3/1
  RMS14/1 -> Scope2/4  "Icir6"
  First-Order Filter2/1 -> Qfuente aux/1
  RMS6/1 -> Scope/4  "Icir2"
  RMS/1 -> Scope/1  "Icli1"
  [ICli1] -> RMS/1  "Icli1"
  [VCir1] -> RMS4/1  "VCir1"
  RMS4/1 -> Tensiones sistema/2  "Vcir1"
  [VR2PRIM] -> RMS5/1  "VR2Prim"
  [ICir6] -> RMS14/1  "Icir6"
  [IAT] -> RMS2/1  "IAT"
  RMS2/1 -> Scope/3  "IAT"
  RMS15/1 -> Scope3/4  "VCir6"
  [ICir3] -> RMS8/1  "Icir3"
  [VCir4] -> RMS12/1  "VCir4"
  [ICir4] -> RMS9/1  "Icir4"
  [VFuenteAux] -> "Power (3ph, Instantaneous)1"/1
  RMS12/1 -> Scope3/2  "VCir4"
  RMS10/1 -> Scope2/3  "Icir5"
  [IFuenteAux] -> "Power (3ph, Instantaneous)1"/2
  RMS11/1 -> Scope3/1  "Vcir3"
  "Power (3ph, Instantaneous)1"/1 -> First-Order Filter1/1
  RMS8/1 -> Scope2/1  "Icir3"
  [IFuenteAux] -> Sequence Analyzer2/1
  Sequence Analyzer2/2 -> Ifuenteaux/2
  Sequence Analyzer1/1 -> Vfuenteaux/1
  [VCli1BT_2] -> Cliente 1 BT2/1, RMS16/1
  [VR1SEC] -> Scope4/1, RMS18/1  "VR1"
  [VR2SEC] -> Scope4/2, RMS19/1  "VR2"
  RMS20/1 -> Bus Creator/2, Scope1/3  "Vcli"
  RMS18/1 -> Scope1/1  "VR1"
  RMS19/1 -> Bus Creator/1, Scope1/2  "VR2"
  [VCli1] -> Scope4/3, RMS20/1  "Vcli"
  Bus Creator/1 -> To Workspace/1
  connections:
  Three-Phase Series RLC Load9/LConn3 -- Distributed Parameters Line15/RConn3
  Three-Phase Transformer Inductance Matrix Type (Two Windings)1/RConn2 -- Three-Phase Series RLC Load2/LConn2
  Three-Phase V-I Measurement10/RConn3 -- Three-Phase Fault/LConn3 -- Distributed Parameters Line11/LConn3
  Three-Phase Transformer Inductance Matrix Type (Two Windings)2/RConn1 -- Three-Phase V-I Measurement3/LConn1
  Three-Phase V-I Measurement5/RConn3 -- Subsystem3/LConn3
  Distributed Parameters Line15/LConn3 -- Distributed Parameters Line11/RConn3 -- Three-Phase Series RLC Load8/LConn3
  Three-Phase V-I Measurement5/LConn2 -- Three-Phase V-I Measurement3/RConn2 -- Three-Phase V-I Measurement9/LConn2 -- Three-Phase V-I Measurement7/LConn2
  Distributed Parameters Line10/RConn2 -- Distributed Parameters Line12/LConn2 -- Three-Phase Series RLC Load7/LConn2
  Three-Phase Source/RConn1 -- Three-Phase V-I Measurement2/LConn1
  Subsystem3/RConn3 -- Three-Phase Series RLC Branch4/LConn3
  Three-Phase V-I Measurement6/LConn2 -- Three-Phase Series RLC Branch2/RConn2
  Three-Phase Series RLC Branch3/RConn2 -- Three-Phase Series RLC Load3/LConn2
  Three-Phase Transformer Inductance Matrix Type (Two Windings)1/RConn3 -- Three-Phase Series RLC Load2/LConn3
  Three-Phase V-I Measurement/LConn2 -- Three-Phase V-I Measurement1/LConn2 -- Three-Phase V-I Measurement2/RConn2
  Three-Phase Series RLC Branch/LConn3 -- Three-Phase Series RLC Branch2/LConn3 -- Three-Phase Series RLC Branch4/RConn3
  Distributed Parameters Line7/RConn1 -- Three-Phase Series RLC Branch3/LConn1 -- Three-Phase Series RLC Load5/LConn1
  Subsystem3/RConn2 -- Three-Phase Series RLC Branch4/LConn2
  Three-Phase V-I Measurement5/RConn1 -- Subsystem3/LConn1
  Distributed Parameters Line17/LConn1 -- Three-Phase V-I Measurement11/RConn1
  Three-Phase Transformer Inductance Matrix Type (Two Windings)4/RConn1 -- Three-Phase V-I Measurement4/LConn1
  Three-Phase V-I Measurement8/RConn3 -- Distributed Parameters Line7/LConn3
  Three-Phase Series RLC Load8/LConn2 -- Distributed Parameters Line11/RConn2 -- Distributed Parameters Line15/LConn2
  Three-Phase V-I Measurement9/RConn3 -- Distributed Parameters Line10/LConn3
  Three-Phase V-I Measurement3/RConn1 -- Three-Phase V-I Measurement9/LConn1 -- Three-Phase V-I Measurement7/LConn1 -- Three-Phase V-I Measurement5/LConn1
  Three-Phase Series RLC Branch3/RConn1 -- Three-Phase Series RLC Load3/LConn1
  Load Flow Bus3/LConn1 -- Three-Phase Transformer Inductance Matrix Type (Two Windings)1/RConn1 -- Three-Phase Series RLC Load2/LConn1
  Three-Phase Series RLC Branch3/RConn3 -- Three-Phase Series RLC Load3/LConn3
  Three-Phase Transformer Inductance Matrix Type (Two Windings)4/LConn1 -- Three-Phase V-I Measurement1/RConn1
  Three-Phase V-I Measurement5/RConn2 -- Subsystem3/LConn2
  Three-Phase V-I Measurement5/LConn3 -- Three-Phase V-I Measurement7/LConn3 -- Three-Phase V-I Measurement9/LConn3 -- Three-Phase V-I Measurement3/RConn3
  Subsystem3/RConn1 -- Three-Phase Series RLC Branch4/LConn1
  Three-Phase Transformer Inductance Matrix Type (Two Windings)4/RConn2 -- Three-Phase V-I Measurement4/LConn2
  Three-Phase Series RLC Branch4/RConn1 -- Three-Phase Series RLC Branch/LConn1 -- Three-Phase Series RLC Branch2/LConn1
  Three-Phase Transformer Inductance Matrix Type (Two Windings)4/RConn3 -- Three-Phase V-I Measurement4/LConn3
  Three-Phase V-I Measurement3/LConn3 -- Three-Phase Transformer Inductance Matrix Type (Two Windings)2/RConn3
  Distributed Parameters Line12/RConn3 -- Distributed Parameters Line21/LConn3
  Three-Phase Series RLC Load1/LConn1 -- Three-Phase Series RLC Branch1/LConn1 -- Three-Phase Series RLC Branch/RConn1
  Distributed Parameters Line10/RConn3 -- Distributed Parameters Line12/LConn3 -- Three-Phase Series RLC Load7/LConn3
  Three-Phase V-I Measurement2/RConn1 -- Load Flow Bus/LConn1 -- Three-Phase V-I Measurement/LConn1 -- Three-Phase V-I Measurement1/LConn1
  Three-Phase Source/RConn2 -- Three-Phase V-I Measurement2/LConn2
  Three-Phase Source/RConn3 -- Three-Phase V-I Measurement2/LConn3
  Three-Phase V-I Measurement4/RConn1 -- Three-Phase V-I Measurement11/LConn1 -- Three-Phase V-I Measurement10/LConn1 -- Three-Phase V-I Measurement8/LConn1
  Distributed Parameters Line21/RConn2 -- Three-Phase Series RLC Load6/LConn2
  Three-Phase Transformer Inductance Matrix Type (Two Windings)2/RConn2 -- Three-Phase V-I Measurement3/LConn2
  Three-Phase Transformer Inductance Matrix Type (Two Windings)4/LConn2 -- Three-Phase V-I Measurement1/RConn2
  Three-Phase Series RLC Load9/LConn2 -- Distributed Parameters Line15/RConn2
  Three-Phase Transformer Inductance Matrix Type (Two Windings)4/LConn3 -- Three-Phase V-I Measurement1/RConn3
  Three-Phase Series RLC Branch/LConn2 -- Three-Phase Series RLC Branch4/RConn2 -- Three-Phase Series RLC Branch2/LConn2
  Three-Phase Series RLC Load1/LConn2 -- Three-Phase Series RLC Branch1/LConn2 -- Three-Phase Series RLC Branch/RConn2
  Three-Phase V-I Measurement6/LConn1 -- Three-Phase Series RLC Branch2/RConn1
  Three-Phase Transformer Inductance Matrix Type (Two Windings)1/LConn2 -- Three-Phase V-I Measurement6/RConn2
  Three-Phase Series RLC Load/LConn1 -- Three-Phase Series RLC Branch1/RConn1
  Three-Phase Transformer Inductance Matrix Type (Two Windings)1/LConn1 -- Three-Phase V-I Measurement6/RConn1
  Three-Phase V-I Measurement6/LConn3 -- Three-Phase Series RLC Branch2/RConn3
  Three-Phase Series RLC Load8/LConn1 -- Distributed Parameters Line11/RConn1 -- Distributed Parameters Line15/LConn1
  Three-Phase V-I Measurement7/RConn1 -- Distributed Parameters Line4/LConn1
  Three-Phase V-I Measurement/LConn3 -- Three-Phase V-I Measurement1/LConn3 -- Three-Phase V-I Measurement2/RConn3
  Three-Phase V-I Measurement7/RConn2 -- Distributed Parameters Line4/LConn2
  Distributed Parameters Line7/RConn2 -- Three-Phase Series RLC Branch3/LConn2 -- Three-Phase Series RLC Load5/LConn2
  Three-Phase V-I Measurement8/RConn1 -- Distributed Parameters Line7/LConn1
  Three-Phase Series RLC Load/LConn2 -- Three-Phase Series RLC Branch1/RConn2
  Three-Phase V-I Measurement9/RConn1 -- Distributed Parameters Line10/LConn1
  Distributed Parameters Line17/LConn3 -- Three-Phase V-I Measurement11/RConn3
  Distributed Parameters Line17/RConn3 -- Three-Phase Series RLC Load10/LConn3
  Three-Phase V-I Measurement8/LConn3 -- Three-Phase V-I Measurement10/LConn3 -- Three-Phase V-I Measurement11/LConn3 -- Three-Phase V-I Measurement4/RConn3
  Three-Phase V-I Measurement9/RConn2 -- Distributed Parameters Line10/LConn2
  Distributed Parameters Line17/LConn2 -- Three-Phase V-I Measurement11/RConn2
  Three-Phase V-I Measurement8/RConn2 -- Distributed Parameters Line7/LConn2
  Three-Phase V-I Measurement10/RConn1 -- Three-Phase Fault/LConn1 -- Distributed Parameters Line11/LConn1
  Distributed Parameters Line11/LConn2 -- Three-Phase Fault/LConn2 -- Three-Phase V-I Measurement10/RConn2
  Distributed Parameters Line12/LConn1 -- Distributed Parameters Line10/RConn1 -- Three-Phase Series RLC Load7/LConn1
  Distributed Parameters Line12/RConn1 -- Distributed Parameters Line21/LConn1
  Distributed Parameters Line12/RConn2 -- Distributed Parameters Line21/LConn2
  Distributed Parameters Line21/RConn3 -- Three-Phase Series RLC Load6/LConn3
  Three-Phase Series RLC Load5/LConn3 -- Distributed Parameters Line7/RConn3 -- Three-Phase Series RLC Branch3/LConn3
  Three-Phase Transformer Inductance Matrix Type (Two Windings)2/LConn3 -- Three-Phase V-I Measurement/RConn3
  Three-Phase Transformer Inductance Matrix Type (Two Windings)2/LConn2 -- Three-Phase V-I Measurement/RConn2
  Three-Phase V-I Measurement8/LConn2 -- Three-Phase V-I Measurement10/LConn2 -- Three-Phase V-I Measurement11/LConn2 -- Three-Phase V-I Measurement4/RConn2
  Three-Phase Series RLC Load/LConn3 -- Three-Phase Series RLC Branch1/RConn3
  Distributed Parameters Line17/RConn1 -- Three-Phase Series RLC Load10/LConn1
  Three-Phase Series RLC Load9/LConn1 -- Distributed Parameters Line15/RConn1
  Three-Phase Series RLC Load4/LConn3 -- Distributed Parameters Line4/RConn3
  Three-Phase Series RLC Load4/LConn2 -- Distributed Parameters Line4/RConn2
  Three-Phase Transformer Inductance Matrix Type (Two Windings)2/LConn1 -- Three-Phase V-I Measurement/RConn1
  Three-Phase V-I Measurement7/RConn3 -- Distributed Parameters Line4/LConn3
  Three-Phase Series RLC Load10/LConn2 -- Distributed Parameters Line17/RConn2
  Three-Phase Transformer Inductance Matrix Type (Two Windings)1/LConn3 -- Three-Phase V-I Measurement6/RConn3
  Three-Phase Series RLC Load4/LConn1 -- Distributed Parameters Line4/RConn1
  Distributed Parameters Line21/RConn1 -- Three-Phase Series RLC Load6/LConn1
  Three-Phase Series RLC Load1/LConn3 -- Three-Phase Series RLC Branch/RConn3 -- Three-Phase Series RLC Branch1/LConn3
